simulink model "Model_hamownika"  (R2024b)
settings: Solver=ode4  StartTime=0.0  StopTime=20  FixedStep=0.01  RelTol=1e-3
undefined symbols (not defined in the file): h, k11, k12, k21, k22, m1, m21, m22, m31, m32
settings Model: Creator=mati  LastModifiedBy=mati

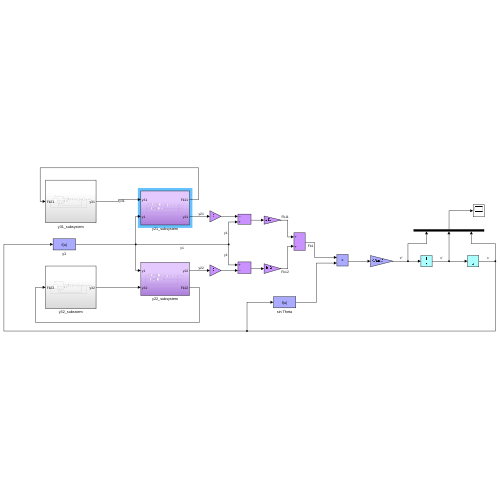
[thumbnail: Simulink's stored preview of the top-level diagram]
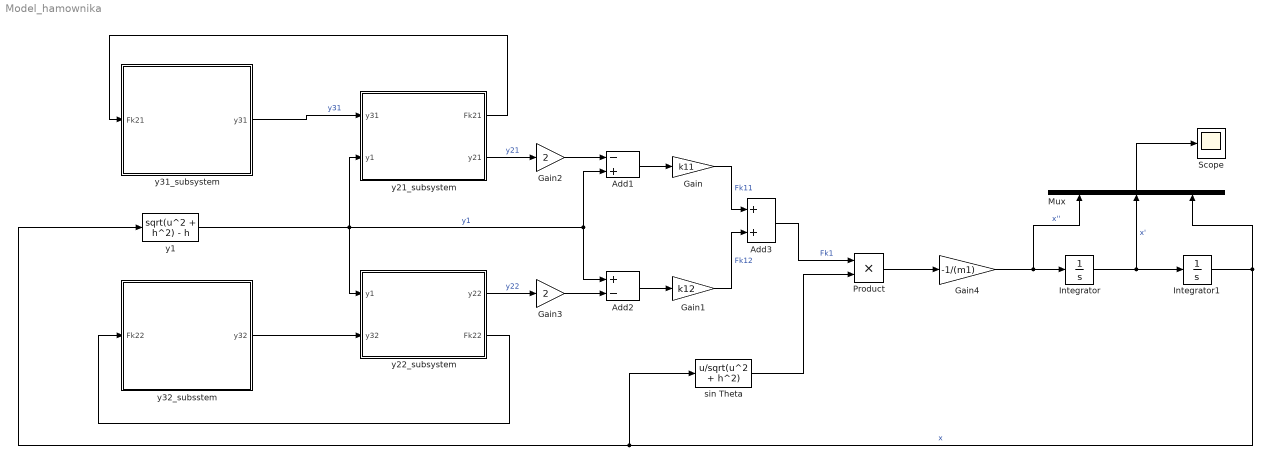
== system Model_hamownika ==
  Add1 : Sum  Inputs=-+
  Add2 : Sum  Inputs=+-
  Add3 : Sum
  Gain : Gain  Gain=k11
  Gain1 : Gain  Gain=k12
  Gain2 : Gain  Gain=2
  Gain3 : Gain  Gain=2
  Gain4 : Gain  Gain=-1/(m1)
  Integrator : Integrator  InitialCondition=67
  Integrator1 : Integrator
  Mux : Mux  Inputs=3
  Product : Product
  Scope : Scope
  sin Theta : Fcn  Expr=u/sqrt(u^2 + h^2)
  y1 : Fcn  Expr=sqrt(u^2 + h^2) - h
  y21_subsystem : Subsystem
  y22_subsystem : Subsystem
  y31_subsystem : Subsystem
  y32_subsstem : Subsystem
  wires:
  Gain4/1 -> Integrator/1, Mux/1  "x''"
  y1/1 -> y21_subsystem/2(y1), Add1/2, Add2/1, y22_subsystem/1(y1)  "y1"
  sin Theta/1 -> Product/2
  Integrator1/1 -> Mux/3, sin Theta/1, y1/1  "x"
  Mux/1 -> Scope/1
  Integrator/1 -> Integrator1/1, Mux/2  "x'"
  Product/1 -> Gain4/1
  Add1/1 -> Gain/1
  Add3/1 -> Product/1  "Fk1"
  y22_subsystem/1(y22) -> Gain3/1  "y22"
  Gain/1 -> Add3/1  "Fk11"
  Add2/1 -> Gain1/1
  Gain1/1 -> Add3/2  "Fk12"
  y21_subsystem/2(y21) -> Gain2/1  "y21"
  Gain2/1 -> Add1/1
  Gain3/1 -> Add2/2
  y31_subsystem/1(y31) -> y21_subsystem/1(y31)  "y31"
  y32_subsstem/1(y32) -> y22_subsystem/2(y32)
  y22_subsystem/2(Fk22) -> y32_subsstem/1(Fk22)
  y21_subsystem/1(Fk21) -> y31_subsystem/1(Fk21)

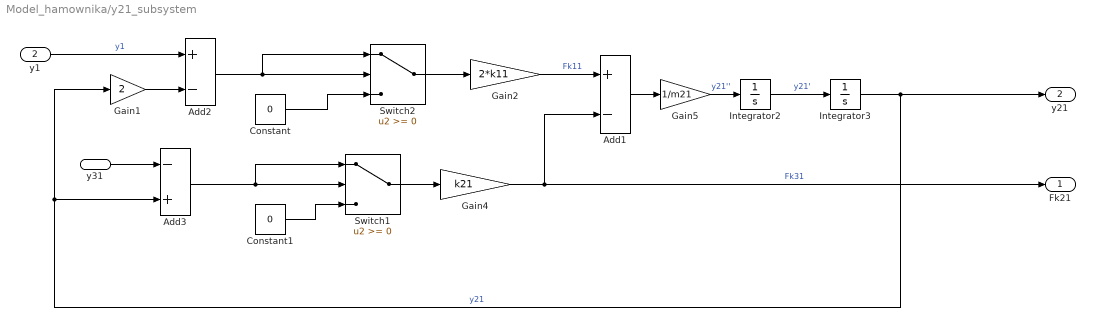
== system Model_hamownika/y21_subsystem ==
  y31 : Inport
  y1 : Inport  Port=2
  Add1 : Sum  Inputs=+-
  Add2 : Sum  Inputs=+-
  Add3 : Sum  Inputs=-+
  Constant : Constant  Value=0
  Constant1 : Constant  Value=0
  Gain1 : Gain  Gain=2
  Gain2 : Gain  Gain=2*k11
  Gain4 : Gain  Gain=k21
  Gain5 : Gain  Gain=1/m21
  Integrator2 : Integrator
  Integrator3 : Integrator
  Switch1 : Switch  SaturateOnIntegerOverflow=off  InputSameDT=off
  Switch2 : Switch  SaturateOnIntegerOverflow=off  InputSameDT=off
  Fk21 : Outport
  y21 : Outport  Port=2
  wires:
  Integrator2/1 -> Integrator3/1  "y21'"
  y1/1 -> Add2/1  "y1"
  Gain2/1 -> Add1/1  "Fk11"
  Gain1/1 -> Add2/2
  Integrator3/1 -> y21/1, Add3/2, Gain1/1  "y21"
  Gain4/1 -> Fk21/1, Add1/2  "Fk31"
  Switch2/1 -> Gain2/1
  Add2/1 -> Switch2/1, Switch2/2
  Constant/1 -> Switch2/3
  Gain5/1 -> Integrator2/1  "y21''"
  Add1/1 -> Gain5/1
  Constant1/1 -> Switch1/3
  Switch1/1 -> Gain4/1
  Add3/1 -> Switch1/1, Switch1/2
  y31/1 -> Add3/1

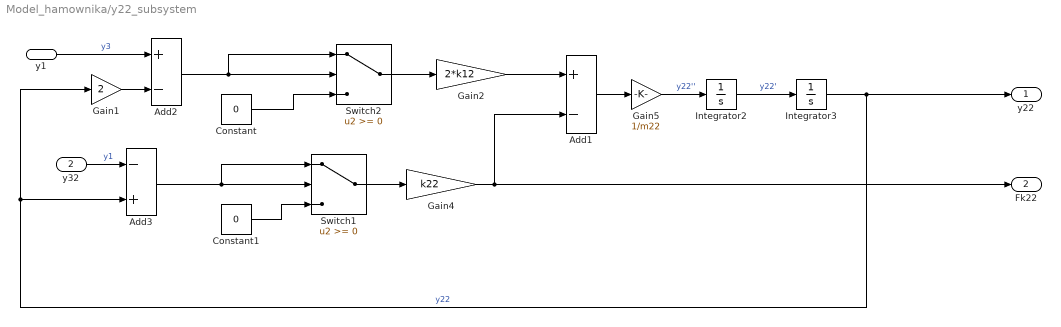
== system Model_hamownika/y22_subsystem ==
  y1 : Inport
  y32 : Inport  Port=2
  Add1 : Sum  Inputs=+-
  Add2 : Sum  Inputs=+-
  Add3 : Sum  Inputs=-+
  Constant : Constant  Value=0
  Constant1 : Constant  Value=0
  Gain1 : Gain  Gain=2
  Gain2 : Gain  Gain=2*k12
  Gain4 : Gain  Gain=k22
  Gain5 : Gain  Gain=1/m22
  Integrator2 : Integrator
  Integrator3 : Integrator
  Switch1 : Switch  SaturateOnIntegerOverflow=off  InputSameDT=off
  Switch2 : Switch  SaturateOnIntegerOverflow=off  InputSameDT=off
  y22 : Outport
  Fk22 : Outport  Port=2
  wires:
  Integrator2/1 -> Integrator3/1  "y22'"
  Gain2/1 -> Add1/1
  Gain1/1 -> Add2/2
  Integrator3/1 -> y22/1, Add3/2, Gain1/1  "y22"
  Gain4/1 -> Fk22/1, Add1/2
  Switch2/1 -> Gain2/1
  Add2/1 -> Switch2/1, Switch2/2
  Constant/1 -> Switch2/3
  Gain5/1 -> Integrator2/1  "y22''"
  Add1/1 -> Gain5/1
  Constant1/1 -> Switch1/3
  Switch1/1 -> Gain4/1
  Add3/1 -> Switch1/1, Switch1/2
  y1/1 -> Add2/1  "y3"
  y32/1 -> Add3/1  "y1"

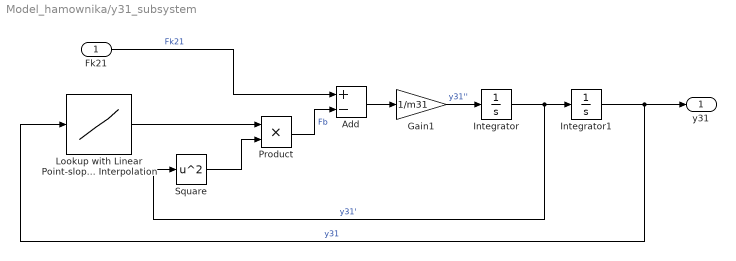
== system Model_hamownika/y31_subsystem ==
  Fk21 : Inport
  Add : Sum  Inputs=+-
  Gain1 : Gain  Gain=1/m31
  Integrator : Integrator
  Integrator1 : Integrator
  Lookup with Linear Point-slope Interpolation : Lookup_n-D  NumberOfTableDimensions=1  BreakpointsForDimension1=[0;10;20;30;40;50;60;70;80;90;94;98;102;104;107;120]  Table=[833;400;160;320;520;520;660;830;1070;1600;2100;2800;4100;5000;9000;9000]  InternalRulePriority=Speed  RndMeth=Simplest
  Product : Product
  Square : Math  Operator=square
  y31 : Outport
  wires:
  Integrator/1 -> Square/1, Integrator1/1  "y31'"
  Integrator1/1 -> Lookup with Linear Point-slope Interpolation/1, y31/1  "y31"
  Add/1 -> Gain1/1
  Fk21/1 -> Add/1  "Fk21"
  Gain1/1 -> Integrator/1  "y31''"
  Square/1 -> Product/2
  Product/1 -> Add/2  "Fb"
  Lookup with Linear Point-slope Interpolation/1 -> Product/1

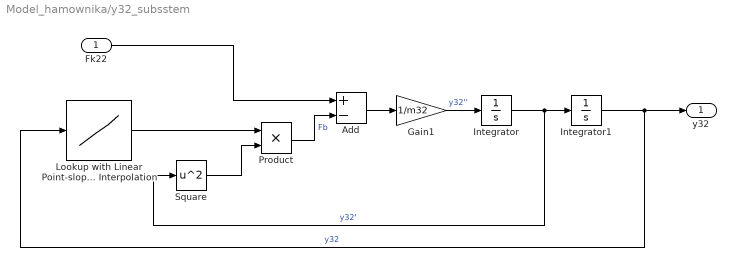
== system Model_hamownika/y32_subsstem ==
  Fk22 : Inport
  Add : Sum  Inputs=+-
  Gain1 : Gain  Gain=1/m32
  Integrator : Integrator
  Integrator1 : Integrator
  Lookup with Linear Point-slope Interpolation : Lookup_n-D  NumberOfTableDimensions=1  BreakpointsForDimension1=[0;10;20;30;40;50;60;70;80;90;94;98;102;104;107;120]  Table=[833;400;160;320;520;520;660;830;1070;1600;2100;2800;4100;5000;9000;9000]  InternalRulePriority=Speed  RndMeth=Simplest
  Product : Product
  Square : Math  Operator=square
  y32 : Outport
  wires:
  Integrator/1 -> Square/1, Integrator1/1  "y32'"
  Integrator1/1 -> Lookup with Linear Point-slope Interpolation/1, y32/1  "y32"
  Add/1 -> Gain1/1
  Gain1/1 -> Integrator/1  "y32''"
  Square/1 -> Product/2
  Product/1 -> Add/2  "Fb"
  Lookup with Linear Point-slope Interpolation/1 -> Product/1
  Fk22/1 -> Add/1
